simulink model "SPH_2022a_new"  (R2022a)
settings: Solver=ode23tb  StartTime=0.0  StopTime=0.02  MaxStep=1E-5  MinStep=1E-6  RelTol=1e-3
libraries: nesl_utility x10, fl_lib x9, ee_lib x5, simulink x1
settings Model: Creator=Kaliamoorthy  LastModifiedBy=HUBERT TONY RAJ
settings ModelReferenceCC: EnableRefExpFcnMdlSchedulingChecks=off
settings RTWCC: Description=Generic Real-Time Target

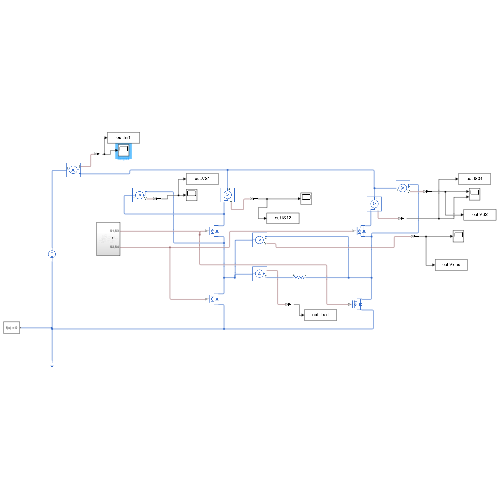
[thumbnail: Simulink's stored preview of the top-level diagram]
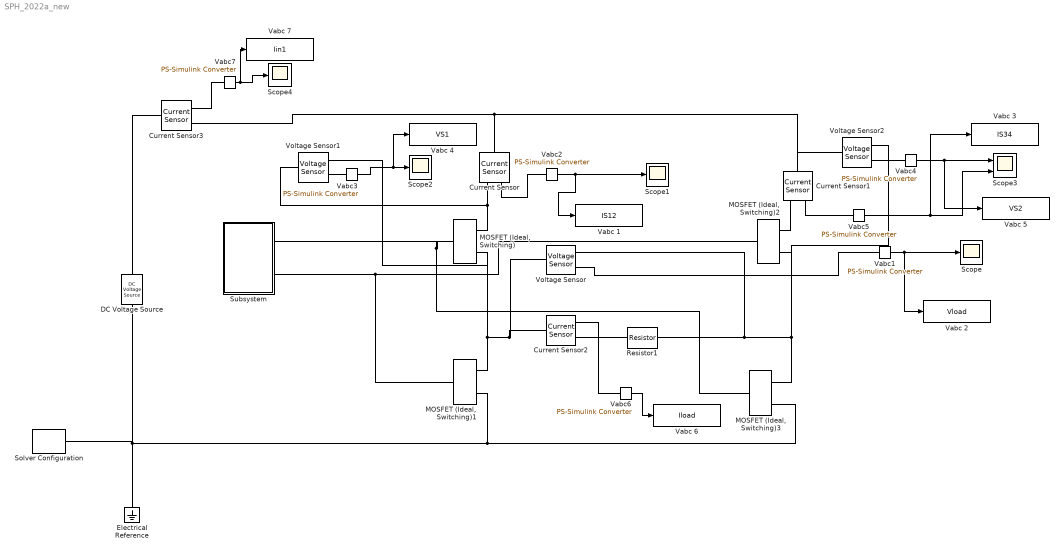
== system SPH_2022a_new ==
  Current Sensor{,1..3} (4 alike) : fl_lib/Electrical/Electrical Sensors/Current Sensor
      settings: SourceProductBaseCode=PW,SS,VE
  DC Voltage Source : fl_lib/Electrical/Electrical Sources/DC Voltage Source  v0=100 V
      settings: SourceProductBaseCode=PW,SS,VE
  Electrical Reference : fl_lib/Electrical/Electrical Elements/Electrical Reference
      settings: SourceProductBaseCode=PW,SS,VE
  MOSFET (Ideal, Switching){,1..3} (4 alike) : ee_lib/Semiconductors & Converters/MOSFET (Ideal, Switching)  Rds=0.01 Ohm  Goff=1e-6 1/Ohm  Vth=2 V  diode_param=ee.enum.converters.protectiondiode.none  diode_Vf=0.8 V  diode_Ron=0.001 Ohm  diode_Goff=1e-5 1/Ohm  diode_C=50e-9 F  diode_iRM=-235 A  diode_iF=300 A  diode_idot=-50 A/us  diode_trr_param=ee.enum.converters.diodeReverseParam.trr_factor  diode_trr_factor=3  diode_trr=15 us  diode_Qrr=1500 s*uA  thermal_loss_option=ee.enum.converters.thermalLossOption.constantvalues  Von_data=[0, 1.1, 1.3, 1.45, 1.75, 2.25, 2.7; 0, 1, 1.15, 1.35, 1.7, 2.35, 3] V  Tj=[298.15, 398.15] K  Iout_data=[0, 10, 50, 100, 200, 400, 600] A  Eon_data=[0, .29, 1.43, 2.86, 5.71, 13.14, 22.86; 0, .57, 2.63, 5.14, 10.29, 20.57, 30.29] * 1e-3 J  Eoff_data=[0, .21, 1.07, 2.14, 4.29, 9.86, 17.14; 0, .43, 1.97, 3.86, 7.71, 15.43, 22.71] * 1e-3 J  Tj_loss=[298.15, 398.15] K  Iout_data_loss=[0, 10, 50, 100, 200, 400, 600] A  Eon_scalar=22.86e-3 J  Eoff_scalar=17.14e-3 J  Voff=300 V  Iout_scalar=600 A  diodeModelType=ee.enum.converters.diodeModelType.pwl  diodeTableType=ee.enum.diode.tableType.IfMat  diode_IfMat=[.07, .12, .19, 1.75, 4.24, 7.32, 11.2; .16, .3, .72, 2.14, 4.02, 6.35, 9.12] A  diode_VfMat=[.9, 1.15, 1.25, 1.5, 1.75, 2.17, 2.6, 2.85; .58, .68, .75, 1.1, 1.38, 1.77, 2.27, 2.7] V  diode_TjVec=[25, 125] degC  diode_VfVec=[.5, .7, .9, 1.3, 1.7, 2.1, 2.5] V  diode_IfVec=[.1, .2, .5, 1, 2, 4, 7, 10] A  diode_Vr=-600 V  diode_Ls=150 nH  diode_Erec=0.03 J  thermal_network_parameterization=ee.enum.thermalNetworkTopology.external  Rth=[.03, .2] K/W  Rth_Cauer=[.03, .1, .2] K/W  Rth_Foster=[.03, .2] K/W  thermal_mass_parameterization=ee.enum.thermalNetwork.timeconstant  thermal_mass=[3, 25] J/K  thermal_mass_Cauer=[3, 10, 25] J/K  thermal_mass_Foster=[33, 50] J/K  thermal_time_constant=[.1, 5] s  thermal_time_constant_Cauer=[.1, 1, 5] s  thermal_time_constant_Foster=[1, 10] s  thermal_mass_initial_temperatures=[25, 25] degC  thermal_mass_initial_temperatures_Cauer=[25, 25, 25] degC  junction_thermal_mass=0.1 J/K  steadyState_Foster=simscape.enum.onoff.on  Tvec_initial_Foster=[25, 25, 25, 25] degC  no_thermal_network=0  junction_temperature_specify=off  junction_temperature_priority=None  junction_temperature=25 degC  junction_temperature_nominal_specify=off  junction_temperature_nominal_unit=degC  junction_temperature_nominal_value=1  vT_specify=off  vT_priority=None  vT=0 V  vT_nominal_specify=off  vT_nominal_unit=V  vT_nominal_value=1  Qj_specify=off  Qj_priority=None  Qj=0 W  Qj_nominal_specify=off  Qj_nominal_unit=W  Qj_nominal_value=1
  Resistor1 : ee_lib/Passive/Resistor  R=50 Ohm  enable_R_tol=0  R_tol=5  tol_distribution=1  nSigma=4  enable_operating_limits=0  operating_limit_action=2  max_working_voltage=100 V  power_rating=1 W  enable_faults=0  fault_action=1  R_faulted=inf Ohm  enable_temporal_fault=0  t_fault=1 s  enable_behavioral_fault=0  max_permissible_current=1 A  t_fail_on_current=1 s  noise_mode=0  sample_time=1e-3 s  repeatability=1  auto_seed=3499211588  user_seed=0  Tdevice=25 degC  power_derating_T1=70 degC  power_derating_T2=155 degC  operating_temperature_range_vec=[-50, 150] degC  alpha=3.93e-3 1/K  Tmeas=25 degC  thermal_mass=100 J/K  temperature_specify=off  temperature_priority=High  temperature=298.15 K  temperature_nominal_specify=off  temperature_nominal_unit=K  temperature_nominal_value=1
  Scope{,1..2,4} (4 alike) : Scope
  Scope3 : Scope  NumInputPorts=2
  Solver Configuration : nesl_utility/Solver Configuration  PhysicalDomain=network_engine_domain  SubClassName=solver  LeftPortType=input  RightPortType=generic  Tones=[]  Harmonics=[]  SimulateNoise=off  Profile=off  UseLocalSampling=off  EnableSwitchedLinearOptims=on  FrequencyDomain=off  UseCCode=off  RelTol=0.001  AbsTol=0.001  MinStep=1e-09  ToWorkspace=off  RevertToSquareIcSolve=off  NumHomotopyIterations=100  PhasorMode=off  PhasorModeNumHarmonics=1  IndexReductionMethod=DerivativeReplacement  DoDC=off  ResidualTolerance=1e-09  UseLocalSolver=off  LocalSolverChoice=NE_BACKWARD_EULER_ADVANCER  LocalSolverSampleTime=0.001  DoFixedCost=off  MaxNonlinIter=3  MaxModeIter=2  ComputeImpulses=off  ImpulseIterations=2  LinearAlgebra=auto  LinearAlgebraNumThread=0  EquationFormulation=NE_TIME_EF  DelaysMemoryBudget=1024  AutomaticFiltering=on  FilteringTimeConstant=0.001  PartitionStorageMethod=AS_NEEDED  PartitionMemoryBudget=1024  PartitionMethod=ROBUST
      settings: SourceProductBaseCode=SS,PW,VE
  Subsystem : Subsystem
  Vabc 1 : ToWorkspace  VariableName=IS12  SaveFormat=Timeseries  SampleTime=-1
  Vabc 2 : ToWorkspace  VariableName=Vload  SaveFormat=Timeseries  SampleTime=-1
  Vabc 3 : ToWorkspace  VariableName=IS34  SaveFormat=Timeseries  SampleTime=-1
  Vabc 4 : ToWorkspace  VariableName=VS1  SaveFormat=Timeseries  SampleTime=-1
  Vabc 5 : ToWorkspace  VariableName=VS2  SaveFormat=Timeseries  SampleTime=-1
  Vabc 6 : ToWorkspace  VariableName=Iload  SaveFormat=Timeseries  SampleTime=-1
  Vabc 7 : ToWorkspace  VariableName=Iin1  SaveFormat=Timeseries  SampleTime=-1
  Vabc{1..7} (7 alike) : nesl_utility/PS-Simulink Converter  PhysicalDomain=network_engine_domain  SubClassName=ps_output  LeftPortType=input  RightPortType=output  PseudoPeriodic=off  Frequencies=[]  VectorFormat=inherit  Unit=inherit  AffineConversion=off
      settings: SourceProductBaseCode=SS,PW,VE
  Voltage Sensor : fl_lib/Electrical/Electrical Sensors/Voltage Sensor
      settings: SourceProductBaseCode=PW,SS,VE
  Voltage Sensor1 : fl_lib/Electrical/Electrical Sensors/Voltage Sensor
      settings: SourceProductBaseCode=PW,SS,VE
  Voltage Sensor2 : fl_lib/Electrical/Electrical Sensors/Voltage Sensor
      settings: SourceProductBaseCode=PW,SS,VE
  wires:
  Vabc1/1 -> Vabc 2/1, Scope/1
  Vabc3/1 -> Vabc 4/1, Scope2/1
  Vabc4/1 -> Vabc 5/1, Scope3/1
  Vabc5/1 -> Vabc 3/1, Scope3/2
  Vabc2/1 -> Vabc 1/1, Scope1/1
  Vabc6/1 -> Vabc 6/1
  Vabc7/1 -> Vabc 7/1, Scope4/1
  connections:
  Voltage Sensor/LConn1 -- Current Sensor2/LConn1 -- "MOSFET (Ideal, Switching)1"/RConn1 -- "MOSFET (Ideal, Switching)"/RConn2 -- Voltage Sensor1/RConn2
  DC Voltage Source/RConn1 -- Solver Configuration/RConn1 -- Electrical Reference/LConn1 -- "MOSFET (Ideal, Switching)1"/RConn2 -- "MOSFET (Ideal, Switching)3"/RConn2
  Voltage Sensor2/LConn1 -- Current Sensor1/LConn1 -- Current Sensor3/RConn2 -- Current Sensor/LConn1
  "MOSFET (Ideal, Switching)3"/RConn1 -- "MOSFET (Ideal, Switching)2"/RConn2 -- Voltage Sensor2/RConn2 -- Resistor1/RConn1 -- Voltage Sensor/RConn2
  Vabc1/LConn1 -- Voltage Sensor/RConn1
  Subsystem/RConn1 -- "MOSFET (Ideal, Switching)3"/LConn1 -- "MOSFET (Ideal, Switching)"/LConn1
  Subsystem/RConn2 -- "MOSFET (Ideal, Switching)1"/LConn1 -- "MOSFET (Ideal, Switching)2"/LConn1
  Current Sensor/RConn2 -- "MOSFET (Ideal, Switching)"/RConn1 -- Voltage Sensor1/LConn1
  Vabc2/LConn1 -- Current Sensor/RConn1
  Vabc3/LConn1 -- Voltage Sensor1/RConn1
  Vabc4/LConn1 -- Voltage Sensor2/RConn1
  "MOSFET (Ideal, Switching)2"/RConn1 -- Current Sensor1/RConn2
  Vabc5/LConn1 -- Current Sensor1/RConn1
  Resistor1/LConn1 -- Current Sensor2/RConn2
  Vabc6/LConn1 -- Current Sensor2/RConn1
  Current Sensor3/LConn1 -- DC Voltage Source/LConn1
  Current Sensor3/RConn1 -- Vabc7/LConn1

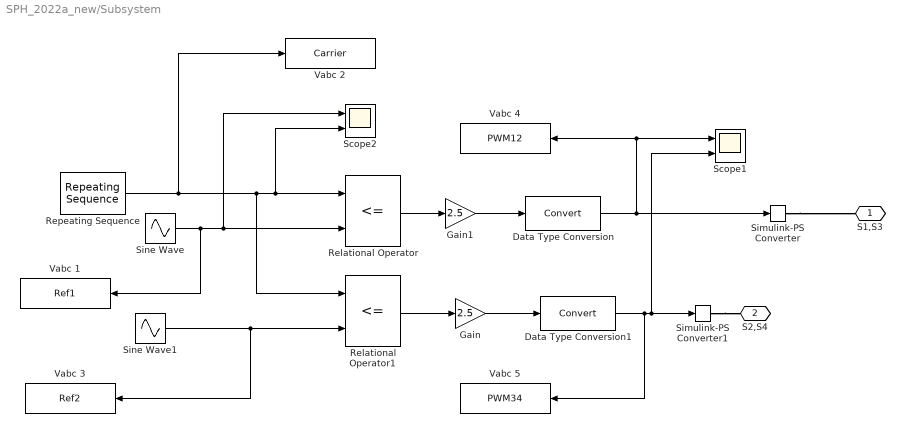
== system SPH_2022a_new/Subsystem ==
  Data Type Conversion : DataTypeConversion  SaturateOnIntegerOverflow=off  RndMeth=Floor
  Data Type Conversion1 : DataTypeConversion  SaturateOnIntegerOverflow=off  RndMeth=Floor
  Gain : Gain  Gain=2.5
  Gain1 : Gain  Gain=2.5
  Relational Operator : RelationalOperator  Operator=<=  OutDataTypeStr=boolean  RndMeth=Simplest  InputSameDT=off
  Relational Operator1 : RelationalOperator  Operator=<=  OutDataTypeStr=boolean  RndMeth=Simplest  InputSameDT=off
  Repeating Sequence : simulink/Sources/Repeating Sequence  rep_seq_t=[0 (1/1250)/2 1/1250]  rep_seq_y=[0 1 0]
  Scope1 : Scope  NumInputPorts=2
  Scope2 : Scope  NumInputPorts=2
  Simulink-PS Converter : nesl_utility/Simulink-PS Converter  PhysicalDomain=network_engine_domain  SubClassName=ps_input  LeftPortType=input  RightPortType=output  PseudoPeriodic=off  Frequencies=[]  NoiseDistribution=none  NoiseParameters=[]  Unit=1  AffineConversion=off  FilteringAndDerivatives=provide  SimscapeFilterOrder=1  InputFilterTimeConstant=0.001  UdotUserProvided=0
      settings: SourceProductBaseCode=SS,PW,VE
  Simulink-PS Converter1 : nesl_utility/Simulink-PS Converter  PhysicalDomain=network_engine_domain  SubClassName=ps_input  LeftPortType=input  RightPortType=output  PseudoPeriodic=off  Frequencies=[]  NoiseDistribution=none  NoiseParameters=[]  Unit=1  AffineConversion=off  FilteringAndDerivatives=provide  SimscapeFilterOrder=1  InputFilterTimeConstant=0.001  UdotUserProvided=0
      settings: SourceProductBaseCode=SS,PW,VE
  Sine Wave : Sin  Amplitude=0.9  Frequency=2*pi*50  SampleTime=0
  Sine Wave1 : Sin  Amplitude=0.9  Frequency=2*pi*50  Phase=pi  SampleTime=0
  Vabc 1 : ToWorkspace  VariableName=Ref1  SaveFormat=Timeseries  SampleTime=-1
  Vabc 2 : ToWorkspace  VariableName=Carrier  SaveFormat=Timeseries  SampleTime=-1
  Vabc 3 : ToWorkspace  VariableName=Ref2  SaveFormat=Timeseries  SampleTime=-1
  Vabc 4 : ToWorkspace  VariableName=PWM12  SaveFormat=Timeseries  SampleTime=-1
  Vabc 5 : ToWorkspace  VariableName=PWM34  SaveFormat=Timeseries  SampleTime=-1
  S1,S3 : PMIOPort  Side=Right
  S2,S4 : PMIOPort  Port=2  Side=Right
  wires:
  Relational Operator/1 -> Gain1/1
  Sine Wave1/1 -> Vabc 3/1, Relational Operator1/2
  Sine Wave/1 -> Vabc 1/1, Scope2/1, Relational Operator/2
  Repeating Sequence/1 -> Vabc 2/1, Relational Operator1/1, Scope2/2, Relational Operator/1
  Relational Operator1/1 -> Gain/1
  Data Type Conversion/1 -> Scope1/1, Vabc 4/1, Simulink-PS Converter/1
  Data Type Conversion1/1 -> Vabc 5/1, Scope1/2, Simulink-PS Converter1/1
  Gain1/1 -> Data Type Conversion/1
  Gain/1 -> Data Type Conversion1/1
  connections:
  Simulink-PS Converter1/RConn1 -- S2,S4/RConn1
  Simulink-PS Converter/RConn1 -- S1,S3/RConn1
